simulink model "Unicycle_Robot_Dynamics_Model"  (R2017b)
settings: Solver=VariableStepAuto  StartTime=0.0  StopTime=10  RelTol=1e-3
settings Model: Creator=Jesus  LastModifiedBy=Jesus

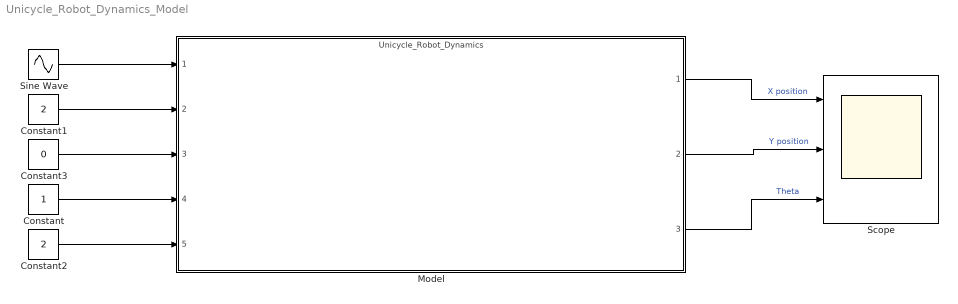
== system Unicycle_Robot_Dynamics_Model ==
  Constant : Constant
  Constant1 : Constant  Value=2
  Constant2 : Constant  Value=2
  Constant3 : Constant  Value=0
  Model : ModelReference  ModelNameDialog=Unicycle_Robot_Dynamics.slx  SimulationMode=Normal  ModelReferenceVersion=1.3
  Scope : Scope  NumInputPorts=3
  Sine Wave : Sin  Frequency=0.01  SampleTime=0
  wires:
  Sine Wave/1 -> Model/1
  Constant/1 -> Model/4
  Constant1/1 -> Model/2
  Constant2/1 -> Model/5
  Constant3/1 -> Model/3
  Model/1 -> Scope/1  "X position"
  Model/2 -> Scope/2  "Y position"
  Model/3 -> Scope/3  "Theta"
